simulink model "HDLRx"  (R2024a)
settings: Solver=FixedStepDiscrete  StartTime=0.0  StopTime=stopTime  RelTol=1e-3
undefined symbols (not defined in the file or in its folder): fPHY, fs, N
libraries: HDL_ieee_8021513 x9, hdlsllib x4, dspsrcs4 x2, whdlutilities x1
settings Model: DataTypeOverride=Off  SimulationMode=accelerator  Creator=cotti  LastModifiedBy=cotti
settings OptimizationCC: BlockReduction=off  ConditionallyExecuteInputs=off  DefaultParameterBehavior=Inlined  InheritOutputTypeSmallerThanSingle=on
settings DebuggingCC: ArtificialAlgebraicLoopMsg=error  SingleTaskRateTransMsg=error
settings HardwareCC: ProdBitPerPointer=32  ProdBitPerSizeT=32  ProdBitPerPtrDiffT=32  ProdLargestAtomicFloat=None  ProdIntDivRoundTo=Undefined  ProdEndianess=Unspecified  ProdWordSize=32  ProdHWDeviceType=ASIC/FPGA->ASIC/FPGA  TargetBitPerLong=64  TargetBitPerPointer=64  TargetBitPerSizeT=64  TargetBitPerPtrDiffT=64  TargetLongLongMode=on  TargetIntDivRoundTo=Zero  TargetEndianess=LittleEndian  TargetWordSize=64  TargetHWDeviceType=Custom Processor->MATLAB Host Computer  ProdEqTarget=off

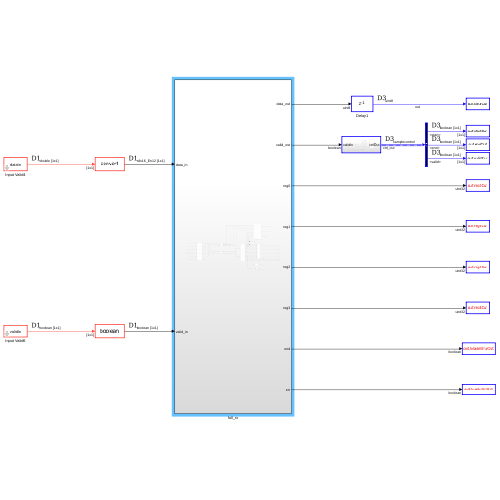
[thumbnail: Simulink's stored preview of the top-level diagram]
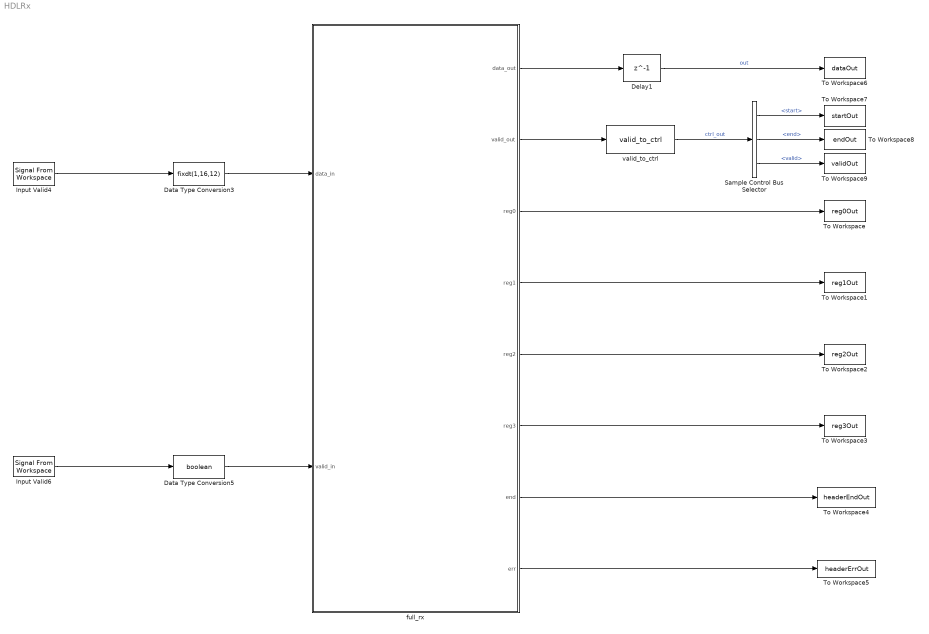
== system HDLRx ==
  Data Type Conversion3 : DataTypeConversion  OutDataTypeStr=fixdt(1,16,12)  SaturateOnIntegerOverflow=off  RndMeth=Floor
  Data Type Conversion5 : DataTypeConversion  OutDataTypeStr=boolean  SaturateOnIntegerOverflow=off  RndMeth=Floor
  Delay1 : Delay  DelayLength=1  InitialCondition=0  UseCircularBuffer=on
  Input Valid4 : dspsrcs4/Signal From Workspace  X=dataIn  Ts=1/fs  nsamps=1  OutputAfterFinalValue=Setting to zero  ignoreOrWarnInputAndFrameLengths=off  OutputFrames=off
  Input Valid6 : dspsrcs4/Signal From Workspace  X=validIn  Ts=1/fs  nsamps=1  OutputAfterFinalValue=Setting to zero  ignoreOrWarnInputAndFrameLengths=off  OutputFrames=off
  Sample Control Bus Selector : whdlutilities/Sample Control Bus Selector  OutputSignals=start,end,valid
  To Workspace : ToWorkspace  VariableName=reg0Out  SampleTime=4/fPHY
      settings: Save2DSignal=2-D array (concatenate along first dimension)
  To Workspace1 : ToWorkspace  VariableName=reg1Out  SampleTime=4/fPHY
      settings: Save2DSignal=2-D array (concatenate along first dimension)
  To Workspace2 : ToWorkspace  VariableName=reg2Out  SampleTime=4/fPHY
      settings: Save2DSignal=2-D array (concatenate along first dimension)
  To Workspace3 : ToWorkspace  VariableName=reg3Out  SampleTime=4/fPHY
      settings: Save2DSignal=2-D array (concatenate along first dimension)
  To Workspace4 : ToWorkspace  VariableName=headerEndOut  SampleTime=4/fPHY
      settings: Save2DSignal=2-D array (concatenate along first dimension)
  To Workspace5 : ToWorkspace  VariableName=headerErrOut  SampleTime=4/fPHY
      settings: Save2DSignal=2-D array (concatenate along first dimension)
  To Workspace6 : ToWorkspace  VariableName=dataOut  SampleTime=4/fPHY
      settings: Save2DSignal=2-D array (concatenate along first dimension)
  To Workspace7 : ToWorkspace  VariableName=startOut  SampleTime=4/fPHY
      settings: Save2DSignal=2-D array (concatenate along first dimension)
  To Workspace8 : ToWorkspace  VariableName=endOut  SampleTime=4/fPHY
      settings: Save2DSignal=2-D array (concatenate along first dimension)
  To Workspace9 : ToWorkspace  VariableName=validOut  SampleTime=4/fPHY
      settings: Save2DSignal=2-D array (concatenate along first dimension)
  full_rx : Subsystem
  valid_to_ctrl : HDL_ieee_8021513/valid_to_ctrl  SystemSampleTime=-1  VariantActivationTime=update diagram  AllowFlexibleInterface=on  Latency=0  AutoFrameSizeCalculation=off
      settings: SourceProductName=HDL IEEE 8021513
  wires:
  Input Valid4/1 -> Data Type Conversion3/1
  Input Valid6/1 -> Data Type Conversion5/1
  Sample Control Bus Selector/3 -> To Workspace9/1  "<valid>"
  Sample Control Bus Selector/2 -> To Workspace8/1  "<end>"
  valid_to_ctrl/1 -> Sample Control Bus Selector/1  "ctrl_out"
  Sample Control Bus Selector/1 -> To Workspace7/1  "<start>"
  Delay1/1 -> To Workspace6/1  "out"
  Data Type Conversion3/1 -> full_rx/1(data_in)
  Data Type Conversion5/1 -> full_rx/2(valid_in)
  full_rx/1(data_out) -> Delay1/1
  full_rx/2(valid_out) -> valid_to_ctrl/1
  full_rx/3(reg0) -> To Workspace/1
  full_rx/4(reg1) -> To Workspace1/1
  full_rx/5(reg2) -> To Workspace2/1
  full_rx/6(reg3) -> To Workspace3/1
  full_rx/7(end) -> To Workspace4/1
  full_rx/8(err) -> To Workspace5/1

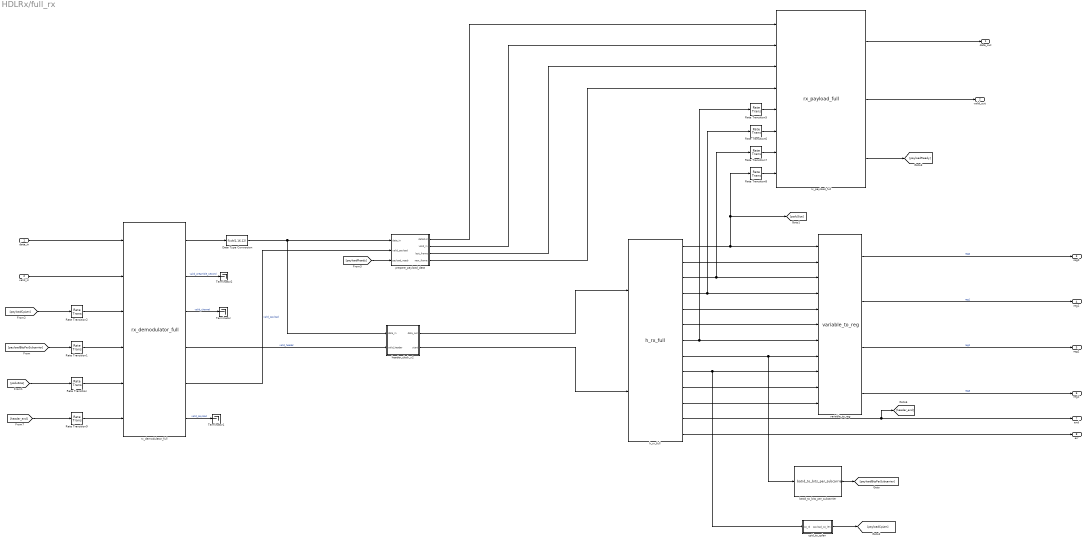
== system HDLRx/full_rx ==
  data_in : Inport
  valid_in : Inport  Port=2
  Data Type Conversion : DataTypeConversion  OutDataTypeStr=fixdt(1,16,12)  SaturateOnIntegerOverflow=off  RndMeth=Floor
  Rate Transition{,1..2,9} (4 alike) : RateTransition  OutPortSampleTime=1/fPHY
  Rate Transition{5..8} (4 alike) : RateTransition  OutPortSampleTime=1/(2*fPHY)
  Terminator : Terminator
  Terminator1 : Terminator
  Terminator2 : Terminator
  batid_to_bits_per_subcarrier : HDL_ieee_8021513/batid_to_bits_per_subcarrier  SystemSampleTime=-1  VariantActivationTime=update diagram  AllowFlexibleInterface=on  Latency=0  AutoFrameSizeCalculation=off
      settings: SourceProductName=HDL IEEE 8021513
  cpid_to_cplen : Subsystem
  h_rx_full : HDL_ieee_8021513/h_rx_full  SystemSampleTime=-1  VariantActivationTime=update diagram  AllowFlexibleInterface=on  Latency=0  AutoFrameSizeCalculation=off
      settings: SourceProductName=HDL IEEE 8021513
  header_clock_x2 : Subsystem
  prepare_payload_data : Subsystem
  rx_demodulator_full : HDL_ieee_8021513/rx_demodulator_full  SystemSampleTime=-1  VariantActivationTime=update diagram  AllowFlexibleInterface=on  Latency=0  AutoFrameSizeCalculation=off
      settings: SourceProductName=HDL IEEE 8021513
  rx_payload_full : HDL_ieee_8021513/rx_payload_full  SystemSampleTime=-1  VariantActivationTime=update diagram  AllowFlexibleInterface=on  Latency=0  AutoFrameSizeCalculation=off
      settings: SourceProductName=HDL IEEE 8021513
  variable_to_reg : HDL_ieee_8021513/variable_to_reg  SystemSampleTime=-1  VariantActivationTime=update diagram  AllowFlexibleInterface=on  Latency=0  AutoFrameSizeCalculation=off
      settings: SourceProductName=HDL IEEE 8021513
  data_out : Outport
  valid_out : Outport  Port=2
  reg0 : Outport  Port=3
  reg1 : Outport  Port=4
  reg2 : Outport  Port=5
  reg3 : Outport  Port=6
  end : Outport  Port=7
  err : Outport  Port=8
  wires:
  h_rx_full/6 -> variable_to_reg/6
  batid_to_bits_per_subcarrier/1 -> [payloadBitsPerSubcarrier]
  Rate Transition7/1 -> rx_payload_full/7
  variable_to_reg/1 -> reg0/1  "reg0"
  Rate Transition2/1 -> rx_demodulator_full/3
  prepare_payload_data/3(last_frame) -> rx_payload_full/3
  header_clock_x2/2(start) -> h_rx_full/2
  rx_demodulator_full/4 -> header_clock_x2/2(valid_header)  "valid_header"
  rx_payload_full/3 -> [payloadReady]
  cpid_to_cplen/1(payload_cp_len) -> [payloadCpLen]
  rx_demodulator_full/3 -> Terminator/1  "valid_channel"
  h_rx_full/10 -> variable_to_reg/10
  Rate Transition5/1 -> rx_payload_full/5
  Rate Transition6/1 -> rx_payload_full/6
  h_rx_full/5 -> variable_to_reg/5
  Rate Transition9/1 -> rx_demodulator_full/6
  data_in/1 -> rx_demodulator_full/1
  h_rx_full/4 -> variable_to_reg/4, Rate Transition6/1
  rx_demodulator_full/1 -> Data Type Conversion/1
  prepare_payload_data/1(dataOut) -> rx_payload_full/1
  h_rx_full/3 -> variable_to_reg/3, Rate Transition7/1
  Data Type Conversion/1 -> prepare_payload_data/1(data_in), header_clock_x2/1(data_in)
  Rate Transition8/1 -> rx_payload_full/8
  h_rx_full/11 -> variable_to_reg/11
  valid_in/1 -> rx_demodulator_full/2
  Rate Transition/1 -> rx_demodulator_full/5
  [payloadReady] -> prepare_payload_data/3(payload_ready)
  rx_payload_full/1 -> data_out/1
  h_rx_full/8 -> batid_to_bits_per_subcarrier/1, variable_to_reg/8
  rx_payload_full/2 -> valid_out/1
  Rate Transition1/1 -> rx_demodulator_full/4
  h_rx_full/1 -> variable_to_reg/1, [psduSize], Rate Transition8/1
  h_rx_full/2 -> variable_to_reg/2
  h_rx_full/9 -> cpid_to_cplen/1(cp_id), variable_to_reg/9
  prepare_payload_data/2(valid_in) -> rx_payload_full/2
  [psduSize] -> Rate Transition/1
  [payloadCpLen] -> Rate Transition2/1
  h_rx_full/13 -> err/1
  prepare_payload_data/4(new_frame) -> rx_payload_full/4
  h_rx_full/7 -> variable_to_reg/7, Rate Transition5/1
  [payloadBitsPerSubcarrier] -> Rate Transition1/1
  rx_demodulator_full/2 -> Terminator2/1  "valid_preamble_second"
  header_clock_x2/1(data_out) -> h_rx_full/1
  variable_to_reg/4 -> reg3/1  "reg3"
  variable_to_reg/2 -> reg1/1  "reg1"
  variable_to_reg/3 -> reg2/1  "reg2"
  h_rx_full/12 -> end/1, [header_end]
  [header_end] -> Rate Transition9/1
  rx_demodulator_full/5 -> prepare_payload_data/2(valid_payload)  "valid_payload"
  rx_demodulator_full/6 -> Terminator1/1  "valid_payload"

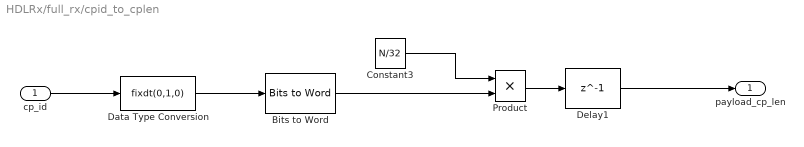
== system HDLRx/full_rx/cpid_to_cplen ==
  cp_id : Inport
  Bits to Word : hdlsllib/Logic and Bit Operations/Bits to Word
  Constant3 : Constant  Value=N/32  OutDataTypeStr=fixdt(0,4,0)  SampleTime=-1
  Data Type Conversion : DataTypeConversion  OutDataTypeStr=fixdt(0,1,0)  SaturateOnIntegerOverflow=off  RndMeth=Floor
  Delay1 : Delay  DelayLength=1  InitialCondition=0  UseCircularBuffer=on
  Product : Product  OutDataTypeStr=uint8
  payload_cp_len : Outport
  wires:
  cp_id/1 -> Data Type Conversion/1
  Data Type Conversion/1 -> Bits to Word/1
  Product/1 -> Delay1/1
  Bits to Word/1 -> Product/2
  Constant3/1 -> Product/1
  Delay1/1 -> payload_cp_len/1

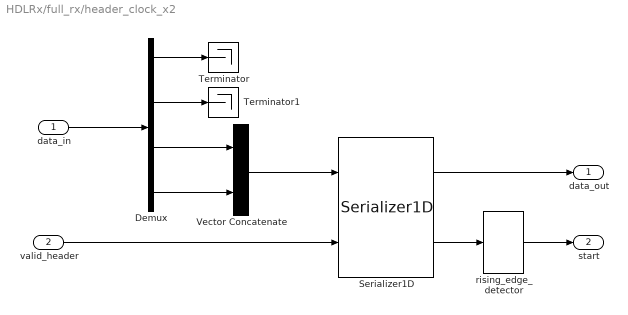
== system HDLRx/full_rx/header_clock_x2 ==
  data_in : Inport
  valid_header : Inport  Port=2
  Demux : Demux
  Serializer1D : hdlsllib/HDL Operations/Serializer1D  Ratio=2  IdleCycles=0  validIn=on  startOut=off  validOut=on  inputDataDimensions=-1  inputSampleTime=-1  inputSignalType=auto
  Terminator : Terminator
  Terminator1 : Terminator
  Vector Concatenate : Concatenate  Mode=Multidimensional array  ConcatenateDimension=2
  rising_edge_detector : HDL_ieee_8021513/rising_edge_detector  SystemSampleTime=-1  VariantActivationTime=update diagram  AllowFlexibleInterface=on  Latency=0  AutoFrameSizeCalculation=off
      settings: SourceProductName=HDL IEEE 8021513
  data_out : Outport
  start : Outport  Port=2
  wires:
  rising_edge_detector/1 -> start/1
  valid_header/1 -> Serializer1D/2
  data_in/1 -> Demux/1
  Demux/1 -> Terminator/1
  Demux/2 -> Terminator1/1
  Demux/3 -> Vector Concatenate/1
  Demux/4 -> Vector Concatenate/2
  Serializer1D/1 -> data_out/1
  Serializer1D/2 -> rising_edge_detector/1
  Vector Concatenate/1 -> Serializer1D/1

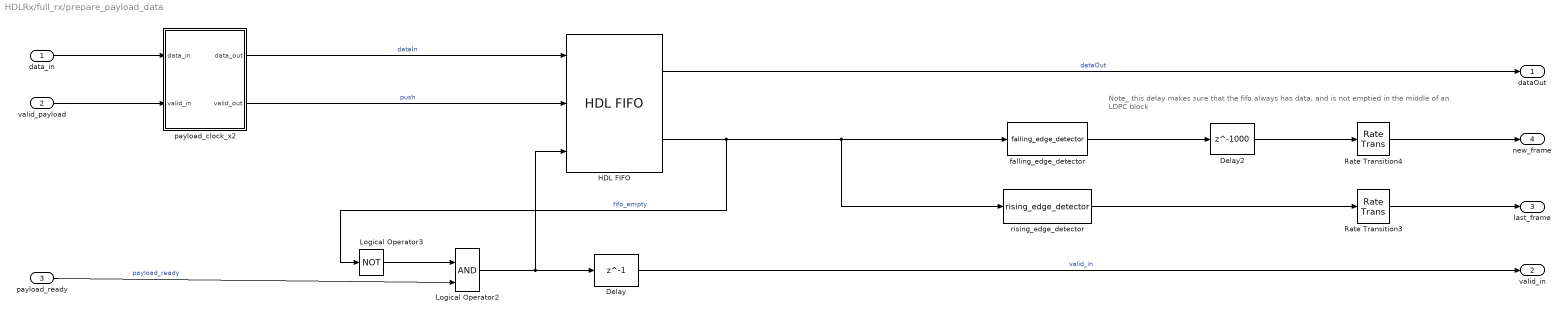
== system HDLRx/full_rx/prepare_payload_data ==
  note: Note_ this delay makes sure that the fifo always has data, and is not emptied in the middle of an LDPC block
  data_in : Inport
  valid_payload : Inport  Port=2
  payload_ready : Inport  Port=3
  Delay : Delay  DelayLength=1  InitialCondition=0  UseCircularBuffer=on
  Delay2 : Delay  DelayLength=1000  InitialCondition=0  UseCircularBuffer=on
  HDL FIFO : hdlsllib/HDL RAMs/HDL FIFO  fifo_size=65536  mode=Classic  ratio=1  push_msg=Error  pop_msg=Error  show_empty=on  show_full=off  show_num=off  LabelModeActiveChoice_Mode=Classic  rst_port=off
  Logical Operator2 : Logic  IconShape=distinctive  AllPortsSameDT=off  OutDataTypeStr=boolean
  Logical Operator3 : Logic  Operator=NOT  IconShape=distinctive  AllPortsSameDT=off  OutDataTypeStr=boolean
  Rate Transition3 : RateTransition  OutPortSampleTime=1/(2*fPHY)
  Rate Transition4 : RateTransition  OutPortSampleTime=1/(2*fPHY)
  falling_edge_detector : HDL_ieee_8021513/falling_edge_detector  SystemSampleTime=-1  VariantActivationTime=update diagram  AllowFlexibleInterface=on  Latency=0  AutoFrameSizeCalculation=off
      settings: SourceProductName=HDL IEEE 8021513
  payload_clock_x2 : Subsystem
  rising_edge_detector : HDL_ieee_8021513/rising_edge_detector  SystemSampleTime=-1  VariantActivationTime=update diagram  AllowFlexibleInterface=on  Latency=0  AutoFrameSizeCalculation=off
      settings: SourceProductName=HDL IEEE 8021513
  dataOut : Outport
  valid_in : Outport  Port=2
  last_frame : Outport  Port=3
  new_frame : Outport  Port=4
  wires:
  data_in/1 -> payload_clock_x2/1(data_in)
  payload_clock_x2/2(valid_out) -> HDL FIFO/2  "push"
  payload_clock_x2/1(data_out) -> HDL FIFO/1  "dataIn"
  HDL FIFO/1 -> dataOut/1  "dataOut"
  valid_payload/1 -> payload_clock_x2/2(valid_in)
  Logical Operator2/1 -> HDL FIFO/3, Delay/1
  Delay/1 -> valid_in/1  "valid_in"
  HDL FIFO/2 -> rising_edge_detector/1, falling_edge_detector/1, Logical Operator3/1  "fifo_empty"
  rising_edge_detector/1 -> Rate Transition3/1
  falling_edge_detector/1 -> Delay2/1
  Delay2/1 -> Rate Transition4/1
  Rate Transition4/1 -> new_frame/1
  Rate Transition3/1 -> last_frame/1
  Logical Operator3/1 -> Logical Operator2/1
  payload_ready/1 -> Logical Operator2/2  "payload_ready"

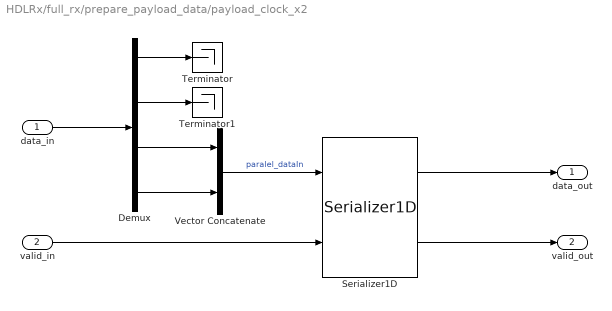
== system HDLRx/full_rx/prepare_payload_data/payload_clock_x2 ==
  data_in : Inport
  valid_in : Inport  Port=2
  Demux : Demux
  Serializer1D : hdlsllib/HDL Operations/Serializer1D  Ratio=2  IdleCycles=0  validIn=on  startOut=off  validOut=on  inputDataDimensions=-1  inputSampleTime=-1  inputSignalType=auto
  Terminator : Terminator
  Terminator1 : Terminator
  Vector Concatenate : Concatenate  Mode=Multidimensional array
  data_out : Outport
  valid_out : Outport  Port=2
  wires:
  Demux/3 -> Vector Concatenate/1
  Demux/1 -> Terminator/1
  data_in/1 -> Demux/1
  Demux/2 -> Terminator1/1
  Serializer1D/1 -> data_out/1
  Serializer1D/2 -> valid_out/1
  valid_in/1 -> Serializer1D/2
  Demux/4 -> Vector Concatenate/2
  Vector Concatenate/1 -> Serializer1D/1  "paralel_dataIn"
